simulink model "condition_action_ex"  (R2022b)
settings: Solver=VariableStepAuto  StartTime=0.0  StopTime=inf  RelTol=1e-3
settings Model: Creator=user  LastModifiedBy=user

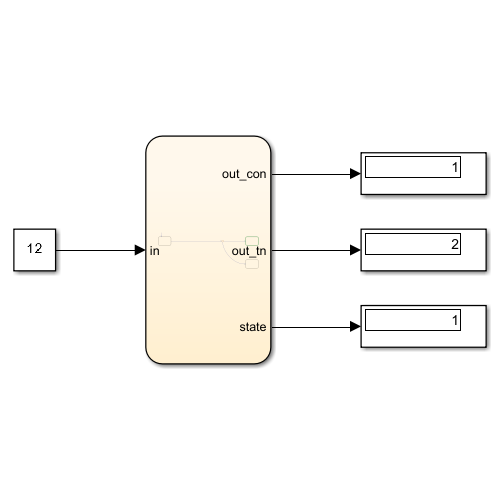
[thumbnail: Simulink's stored preview of the top-level diagram]
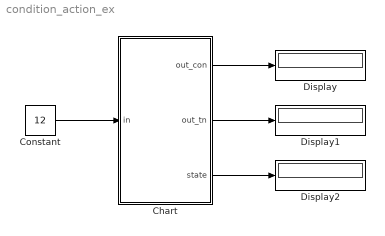
== system condition_action_ex ==
  Chart : Stateflow chart  TreatAsAtomicUnit=on
  Constant : Constant  Value=12
  Display : Display
  Display1 : Display
  Display2 : Display
  wires:
  Chart/1(out_con) -> Display/1
  Chart/3(state) -> Display2/1
  Chart/2(out_tn) -> Display1/1
  Constant/1 -> Chart/1(in)

== stateflow chart condition_action_ex/Chart ==
  state B
    state = 1;
  state A
    state = 0;
  state C
    state = 2;
  (default) -> A
  A -> (junction 5) : [in>0]{out_con = 2;} / {out_con = 1; out_tn = 2;}
  (junction 5) -> B [order 1] : [in>10]
  (junction 5) -> C [order 2] : [in>5]
  data: out_con output; out_tn output; state output; in input
